simulink model "pid_basic_learning"  (R2026a)
settings: Solver=VariableStepAuto
settings Model: Creator=adviksharma  LastModifiedBy=adviksharma

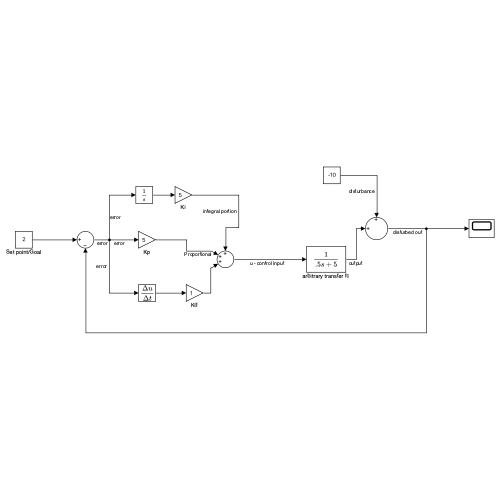
[thumbnail: Simulink's stored preview of the top-level diagram]
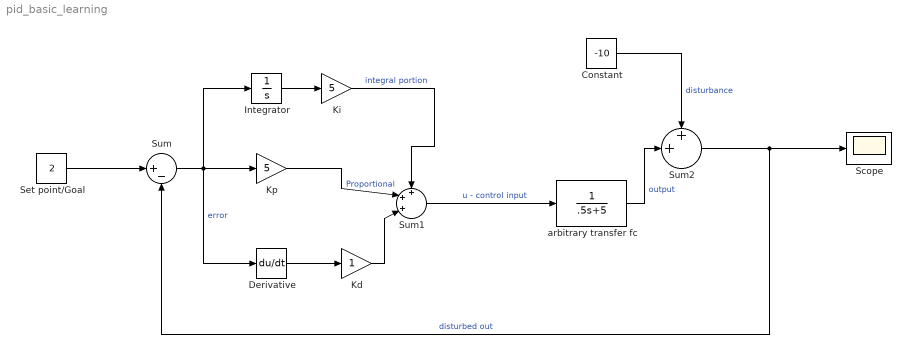
== system pid_basic_learning ==
  Constant : Constant  Value=-10
  Derivative : Derivative
  Integrator : Integrator
  Kd : Gain
  Ki : Gain  Gain=5
  Kp : Gain  Gain=5
  Scope : Scope
      settings: ActiveDisplayYMinimum=-20.793231483461661  ActiveDisplayYMaximum=13.249955620645913
  Set point/Goal : Constant  Value=2
  Sum : Sum  Inputs=|+-
  Sum1 : Sum  Inputs=+++|
  Sum2 : Sum  Inputs=++|
  arbitrary transfer fc : TransferFcn  Denominator=[.5 5]
  wires:
  Set point/Goal/1 -> Sum/1
  Sum/1 -> Derivative/1, Integrator/1, Kp/1  "error"
  Sum1/1 -> arbitrary transfer fc/1  "u - control input"
  Kp/1 -> Sum1/2  "Proportional"
  Integrator/1 -> Ki/1
  Ki/1 -> Sum1/1  "integral portion"
  Derivative/1 -> Kd/1
  Kd/1 -> Sum1/3
  Constant/1 -> Sum2/1  "disturbance"
  arbitrary transfer fc/1 -> Sum2/2  "output"
  Sum2/1 -> Sum/2, Scope/1  "disturbed out"
